simulink model "test_synchronous_machines_EMT_Phasor"  (R2025b)
settings: Solver=VariableStepAuto  StartTime=0.0  StopTime=20  RelTol=1e-3
undefined symbols (not defined in the file): Circuit, DiscIntNeverNeededParam, Open, Short
libraries: fl_lib x6, ee_lib_for_power_systems x6, ee_lib x6, nesl_utility x3
settings Model: Creator=gdudgeon  LastModifiedBy=gdudgeon
settings RTWCC: GPUComputeCapability=3.5

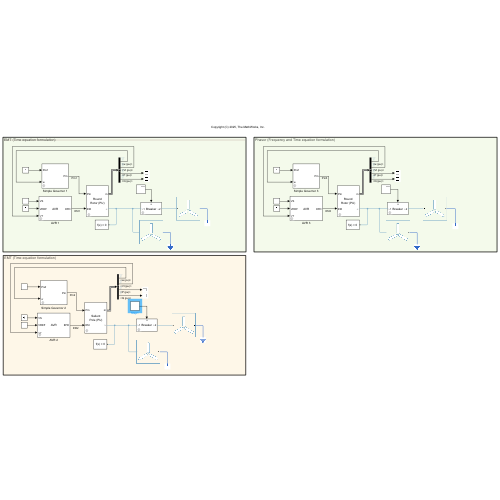
[thumbnail: Simulink's stored preview of the top-level diagram]
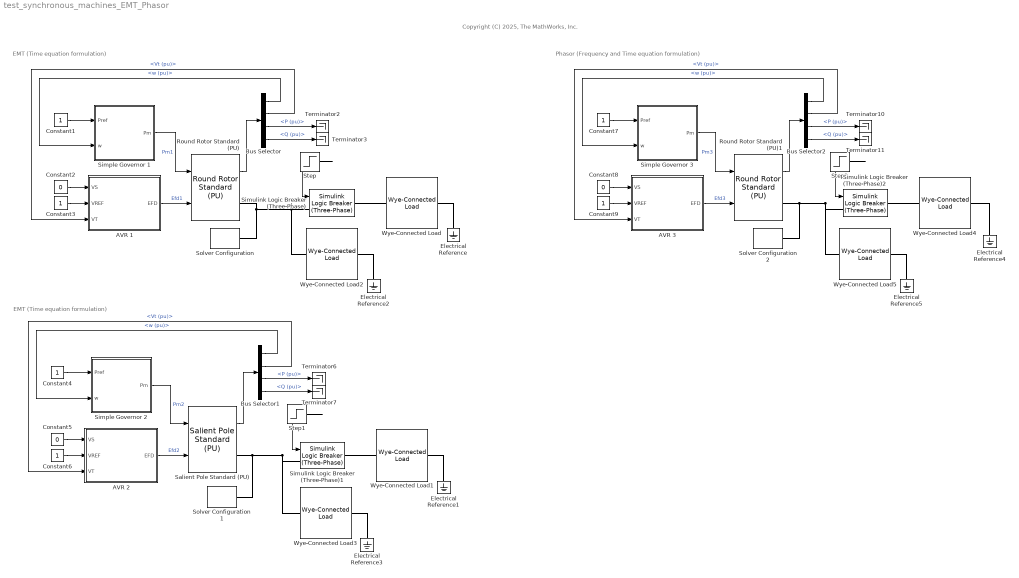
== system test_synchronous_machines_EMT_Phasor ==
  note: EMT (Time equation formulation)
  note: EMT (Time equation formulation)
  note: Phasor (Frequency and Time equation formulation)
  note: Copyright (C) 2025, The MathWorks, Inc.
  AVR 1 : Subsystem  mask{K=200, TE=0.05, EMIN=0, EMAX=4}
      mask Display: disp('AVR')
  AVR 2 : Subsystem  mask{K=200, TE=0.05, EMIN=0, EMAX=4}
      mask Display: disp('AVR')
  AVR 3 : Subsystem  mask{K=200, TE=0.05, EMIN=0, EMAX=4}
      mask Display: disp('AVR')
  Bus Selector : BusSelector  OutputSignals=w (pu),Vt (pu),P (pu),Q (pu)
  Bus Selector1 : BusSelector  OutputSignals=w (pu),Vt (pu),P (pu),Q (pu)
  Bus Selector2 : BusSelector  OutputSignals=w (pu),Vt (pu),P (pu),Q (pu)
  Constant{1,3..4,6..7,9} (6 alike) : Constant
  Constant2 : Constant  Value=0
  Constant5 : Constant  Value=0
  Constant8 : Constant  Value=0
  Electrical Reference{,1..5} (6 alike) : fl_lib/Electrical/Electrical Elements/Electrical Reference
  Round Rotor Standard (PU) : ee_lib_for_power_systems/Electromechanical Machines/Round Rotor Standard (PU)  Pnom=1e6  Vnom=20e3  Fnom=60  Xd=1.5  Xdp=0.4  Xdpp=0.25  Xq=1.4  Xqp=0.5  Xqpp=0.25  Xl=0.1  Ra=0.05  D_Q=[Short-Circuit Open-Circuit]  Tdp=1.2  Tdpp=0.05  Tdop=7  Tdopp=0.05  Tqp=1  Tqpp=0.05  Tqop=1  Tqopp=0.04  H=0.2  D=0  p=4
  Round Rotor Standard (PU)1 : ee_lib_for_power_systems/Electromechanical Machines/Round Rotor Standard (PU)  Pnom=1e6  Vnom=20e3  Fnom=60  Xd=1.5  Xdp=0.4  Xdpp=0.25  Xq=1.4  Xqp=0.5  Xqpp=0.25  Xl=0.1  Ra=0.05  D_Q=[Short-Circuit Open-Circuit]  Tdp=1.2  Tdpp=0.05  Tdop=7  Tdopp=0.05  Tqp=1  Tqpp=0.05  Tqop=1  Tqopp=0.04  H=0.2  D=0  p=4
  Salient Pole Standard (PU) : ee_lib_for_power_systems/Electromechanical Machines/Salient Pole Standard (PU)  Pnom=1e6  Vnom=20e3  Fnom=60  Xd=1.5  Xdp=0.4  Xdpp=0.25  Xq=1.4  Xqpp=0.25  Xl=0.1  Ra=0.05  D_Q=[Short-Circuit Open-Circuit]  Tdp=1.2  Tdpp=0.05  Tdop=7  Tdopp=0.05  Tqpp=0.05  Tqopp=0.04  H=0.2  D=0  p=4
  Simple Governor 1 : Subsystem  mask{R=0.05, T1=0.5, P_MAX=2, P_MIN=0}
  Simple Governor 2 : Subsystem  mask{R=0.05, T1=0.5, P_MAX=2, P_MIN=0}
  Simple Governor 3 : Subsystem  mask{R=0.05, T1=0.5, P_MAX=2, P_MIN=0}
  Simulink Logic Breaker (Three-Phase) : ee_lib_for_power_systems/Network Components/Simulink Logic Breaker (Three-Phase)  initB=1  Ron=1e-6  Goff=1e-6  Ts=5e-5
  Simulink Logic Breaker (Three-Phase)1 : ee_lib_for_power_systems/Network Components/Simulink Logic Breaker (Three-Phase)  initB=1  Ron=1e-6  Goff=1e-6  Ts=5e-5
  Simulink Logic Breaker (Three-Phase)2 : ee_lib_for_power_systems/Network Components/Simulink Logic Breaker (Three-Phase)  initB=1  Ron=1e-6  Goff=1e-6  Ts=5e-5
  "Solver Configuration " : nesl_utility/Solver Configuration  PhysicalDomain=network_engine_domain  SubClassName=solver  LeftPortType=input  RightPortType=generic  Tones=[]  Harmonics=[]  SimulateNoise=off  Profile=off  UseLocalSampling=off  EnableSwitchedLinearOptims=on  FrequencyDomain=off  UseCCode=off  RelTol=0.001  AbsTol=0.001  MinStep=1e-09  ToWorkspace=off  RevertToSquareIcSolve=off  NumHomotopyIterations=100  PhasorMode=off  PhasorModeNumHarmonics=1  ConsistencySolver=NEWTON_XTOL_AFTER_FTOL  IndexReductionMethod=None  DoDC=off  ResidualTolerance=1e-09  ConsistencyTolSource=GLOBAL  ConsistencyAbsTol=0.001  ConsistencyRelTol=0.001  ConsistencyTolFactor=0.001  UseLocalSolver=on  LocalSolverChoice=NE_PARTITIONING_ADVANCER  ResolveIndetEquations=off  FunctionEvalNumThread=1  LocalSolverSampleTime=50e-6  DoFixedCost=off  MaxNonlinIter=2  MaxModeIter=2  ComputeImpulses=off  ImpulseIterations=2  LinearAlgebra=Sparse  LinearAlgebraNumThread=0  EquationFormulation=NE_TIME_EF  DelaysMemoryBudget=1024  AutomaticFiltering=off  FilteringTimeConstant=0.001  PartitionStorageMethod=AS_NEEDED  PartitionMemoryBudget=1024  PartitionMethod=ROBUST  MultibodyUseLocalSolver=off  MultibodyLocalSolverChoice=ODE1  MultibodyLocalSolverSampleTime=0.001
  Solver Configuration 1 : nesl_utility/Solver Configuration  PhysicalDomain=network_engine_domain  SubClassName=solver  LeftPortType=input  RightPortType=generic  Tones=[]  Harmonics=[]  SimulateNoise=off  Profile=off  UseLocalSampling=off  EnableSwitchedLinearOptims=on  FrequencyDomain=off  UseCCode=off  RelTol=0.001  AbsTol=0.001  MinStep=1e-09  ToWorkspace=off  RevertToSquareIcSolve=off  NumHomotopyIterations=100  PhasorMode=off  PhasorModeNumHarmonics=1  ConsistencySolver=NEWTON_XTOL_AFTER_FTOL  IndexReductionMethod=None  DoDC=off  ResidualTolerance=1e-09  ConsistencyTolSource=GLOBAL  ConsistencyAbsTol=0.001  ConsistencyRelTol=0.001  ConsistencyTolFactor=0.001  UseLocalSolver=on  LocalSolverChoice=NE_PARTITIONING_ADVANCER  ResolveIndetEquations=off  FunctionEvalNumThread=1  LocalSolverSampleTime=50e-6  DoFixedCost=off  MaxNonlinIter=2  MaxModeIter=2  ComputeImpulses=off  ImpulseIterations=2  LinearAlgebra=Sparse  LinearAlgebraNumThread=0  EquationFormulation=NE_TIME_EF  DelaysMemoryBudget=1024  AutomaticFiltering=off  FilteringTimeConstant=0.001  PartitionStorageMethod=AS_NEEDED  PartitionMemoryBudget=1024  PartitionMethod=ROBUST  MultibodyUseLocalSolver=off  MultibodyLocalSolverChoice=ODE1  MultibodyLocalSolverSampleTime=0.001
  Solver Configuration 2 : nesl_utility/Solver Configuration  PhysicalDomain=network_engine_domain  SubClassName=solver  LeftPortType=input  RightPortType=generic  Tones=[]  Harmonics=[]  SimulateNoise=off  Profile=off  UseLocalSampling=off  EnableSwitchedLinearOptims=on  FrequencyDomain=off  UseCCode=off  RelTol=0.001  AbsTol=0.001  MinStep=1e-09  ToWorkspace=off  RevertToSquareIcSolve=off  NumHomotopyIterations=100  PhasorMode=off  PhasorModeNumHarmonics=1  ConsistencySolver=NEWTON_XTOL_AFTER_FTOL  IndexReductionMethod=None  DoDC=off  ResidualTolerance=1e-09  ConsistencyTolSource=GLOBAL  ConsistencyAbsTol=0.001  ConsistencyRelTol=0.001  ConsistencyTolFactor=0.001  UseLocalSolver=on  LocalSolverChoice=NE_BACKWARD_EULER_ADVANCER  ResolveIndetEquations=off  FunctionEvalNumThread=1  LocalSolverSampleTime=1/120  DoFixedCost=on  MaxNonlinIter=2  MaxModeIter=2  ComputeImpulses=off  ImpulseIterations=2  LinearAlgebra=auto  LinearAlgebraNumThread=0  EquationFormulation=NE_FREQUENCY_TIME_EF  DelaysMemoryBudget=1024  AutomaticFiltering=off  FilteringTimeConstant=0.001  PartitionStorageMethod=AS_NEEDED  PartitionMemoryBudget=1024  PartitionMethod=ROBUST  MultibodyUseLocalSolver=off  MultibodyLocalSolverChoice=ODE1  MultibodyLocalSolverSampleTime=0.001
  Step : Step  Time=10  SampleTime=5e-5
  Step1 : Step  Time=10  SampleTime=5e-5
  Step2 : Step  Time=10  SampleTime=5e-5
  Terminator{2..3,6..7,10..11} (6 alike) : Terminator
  Wye-Connected Load{,1..5} (6 alike) : ee_lib/Passive/RLC Assemblies/Wye-Connected Load  port_option=ee.enum.threePhasePort.composite  parameterization=ee.enum.rlc.parameterization.ratedpower  component_structure=ee.enum.rlc.structure.R  component_structure_PQ=ee.enum.rlc.structure.R  R=1 Ohm  L=1e-3 H  C=1e-6 F  VRated=20e3 V  FRated=60 Hz  P=5e5 W  Qpos=3e5 A*V  Qneg=-1e2 A*V  R_parasitic=0 Ohm  G_parasitic=0 1/Ohm  R_parasitic_PQ=0 Ohm  G_parasitic_PQ=0 1/Ohm  Vmag0=24e3 V  Vang0=0 deg  Freq0=60 Hz  IL_specify=off  IL_priority=High  IL=[0, 0, 0] A  IL_nominal_specify=off  IL_nominal_value=1  IL_nominal_unit=A  VC_specify=off  VC_priority=High  VC=[0, 0, 0] V  VC_nominal_specify=off  VC_nominal_value=1  VC_nominal_unit=V
  wires:
  Round Rotor Standard (PU)/1 -> Bus Selector/1
  AVR 1/1(EFD) -> Round Rotor Standard (PU)/2  "Efd1"
  Simple Governor 1/1(Pm) -> Round Rotor Standard (PU)/1  "Pm1"
  Step/1 -> Simulink Logic Breaker (Three-Phase)/1
  Bus Selector/1 -> Simple Governor 1/2(w)  "<w (pu)>"
  Constant1/1 -> Simple Governor 1/1(Pref)
  Bus Selector/2 -> AVR 1/3(VT)  "<Vt (pu)>"
  Constant3/1 -> AVR 1/2(VREF)
  Constant2/1 -> AVR 1/1(VS)
  Bus Selector/3 -> Terminator2/1  "<P (pu)>"
  Bus Selector/4 -> Terminator3/1  "<Q (pu)>"
  Bus Selector1/4 -> Terminator7/1  "<Q (pu)>"
  Bus Selector1/3 -> Terminator6/1  "<P (pu)>"
  Constant5/1 -> AVR 2/1(VS)
  Constant6/1 -> AVR 2/2(VREF)
  Bus Selector1/2 -> AVR 2/3(VT)  "<Vt (pu)>"
  Constant4/1 -> Simple Governor 2/1(Pref)
  Bus Selector1/1 -> Simple Governor 2/2(w)  "<w (pu)>"
  Step1/1 -> Simulink Logic Breaker (Three-Phase)1/1
  Simple Governor 2/1(Pm) -> Salient Pole Standard (PU)/1  "Pm2"
  AVR 2/1(EFD) -> Salient Pole Standard (PU)/2  "Efd2"
  Salient Pole Standard (PU)/1 -> Bus Selector1/1
  Bus Selector2/4 -> Terminator11/1  "<Q (pu)>"
  Bus Selector2/3 -> Terminator10/1  "<P (pu)>"
  Constant8/1 -> AVR 3/1(VS)
  Constant9/1 -> AVR 3/2(VREF)
  Bus Selector2/2 -> AVR 3/3(VT)  "<Vt (pu)>"
  Constant7/1 -> Simple Governor 3/1(Pref)
  Bus Selector2/1 -> Simple Governor 3/2(w)  "<w (pu)>"
  Simple Governor 3/1(Pm) -> Round Rotor Standard (PU)1/1  "Pm3"
  AVR 3/1(EFD) -> Round Rotor Standard (PU)1/2  "Efd3"
  Round Rotor Standard (PU)1/1 -> Bus Selector2/1
  Step2/1 -> Simulink Logic Breaker (Three-Phase)2/1
  connections:
  Simulink Logic Breaker (Three-Phase)/LConn1 -- Round Rotor Standard (PU)/RConn1 -- "Solver Configuration "/RConn1 -- Wye-Connected Load2/LConn1
  Electrical Reference/LConn1 -- Wye-Connected Load/RConn1
  Simulink Logic Breaker (Three-Phase)/RConn1 -- Wye-Connected Load/LConn1
  Simulink Logic Breaker (Three-Phase)1/RConn1 -- Wye-Connected Load1/LConn1
  Electrical Reference1/LConn1 -- Wye-Connected Load1/RConn1
  Solver Configuration 1/RConn1 -- Simulink Logic Breaker (Three-Phase)1/LConn1 -- Wye-Connected Load3/LConn1 -- Salient Pole Standard (PU)/RConn1
  Electrical Reference2/LConn1 -- Wye-Connected Load2/RConn1
  Electrical Reference3/LConn1 -- Wye-Connected Load3/RConn1
  Electrical Reference5/LConn1 -- Wye-Connected Load5/RConn1
  Electrical Reference4/LConn1 -- Wye-Connected Load4/RConn1
  Simulink Logic Breaker (Three-Phase)2/RConn1 -- Wye-Connected Load4/LConn1
  Round Rotor Standard (PU)1/RConn1 -- Solver Configuration 2/RConn1 -- Simulink Logic Breaker (Three-Phase)2/LConn1 -- Wye-Connected Load5/LConn1

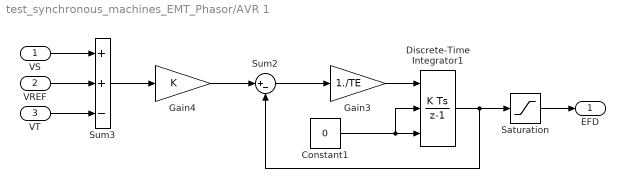
== system test_synchronous_machines_EMT_Phasor/AVR 1 ==
  VS : Inport
  VREF : Inport  Port=2
  VT : Inport  Port=3
  Constant1 : Constant  Value=0  SampleTime=-1
  Discrete-Time Integrator1 : DiscreteIntegrator  ExternalReset=rising  InitialConditionSource=external  SampleTime=-1  UpperSaturationLimit=EMAX  LowerSaturationLimit=EMIN  ICPrevOutput=DiscIntNeverNeededParam  ICPrevScaledInput=DiscIntNeverNeededParam
  Gain3 : Gain  Gain=1./TE
  Gain4 : Gain  Gain=K
  Saturation : Saturate  UpperLimit=EMAX  LowerLimit=EMIN
  Sum2 : Sum  Inputs=|+-
  Sum3 : Sum  Inputs=++-
  EFD : Outport
  wires:
  Sum3/1 -> Gain4/1
  Discrete-Time Integrator1/1 -> Saturation/1, Sum2/2
  Constant1/1 -> Discrete-Time Integrator1/2, Discrete-Time Integrator1/3
  Gain3/1 -> Discrete-Time Integrator1/1
  Sum2/1 -> Gain3/1
  Gain4/1 -> Sum2/1
  VT/1 -> Sum3/3
  VREF/1 -> Sum3/2
  VS/1 -> Sum3/1
  Saturation/1 -> EFD/1

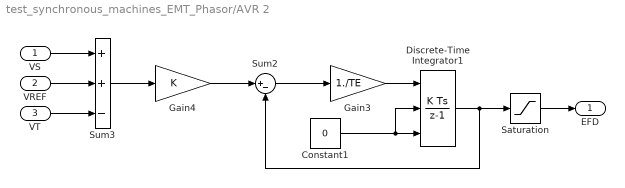
== system test_synchronous_machines_EMT_Phasor/AVR 2 ==
  VS : Inport
  VREF : Inport  Port=2
  VT : Inport  Port=3
  Constant1 : Constant  Value=0  SampleTime=-1
  Discrete-Time Integrator1 : DiscreteIntegrator  ExternalReset=rising  InitialConditionSource=external  SampleTime=-1  UpperSaturationLimit=EMAX  LowerSaturationLimit=EMIN  ICPrevOutput=DiscIntNeverNeededParam  ICPrevScaledInput=DiscIntNeverNeededParam
  Gain3 : Gain  Gain=1./TE
  Gain4 : Gain  Gain=K
  Saturation : Saturate  UpperLimit=EMAX  LowerLimit=EMIN
  Sum2 : Sum  Inputs=|+-
  Sum3 : Sum  Inputs=++-
  EFD : Outport
  wires:
  Saturation/1 -> EFD/1
  VS/1 -> Sum3/1
  VREF/1 -> Sum3/2
  VT/1 -> Sum3/3
  Gain4/1 -> Sum2/1
  Sum2/1 -> Gain3/1
  Gain3/1 -> Discrete-Time Integrator1/1
  Constant1/1 -> Discrete-Time Integrator1/3, Discrete-Time Integrator1/2
  Discrete-Time Integrator1/1 -> Sum2/2, Saturation/1
  Sum3/1 -> Gain4/1

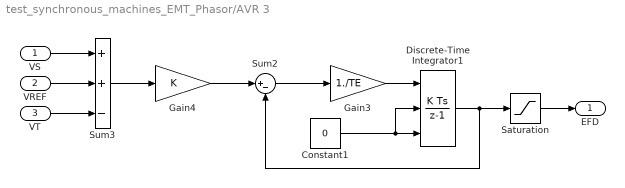
== system test_synchronous_machines_EMT_Phasor/AVR 3 ==
  VS : Inport
  VREF : Inport  Port=2
  VT : Inport  Port=3
  Constant1 : Constant  Value=0  SampleTime=-1
  Discrete-Time Integrator1 : DiscreteIntegrator  ExternalReset=rising  InitialConditionSource=external  SampleTime=-1  UpperSaturationLimit=EMAX  LowerSaturationLimit=EMIN  ICPrevOutput=DiscIntNeverNeededParam  ICPrevScaledInput=DiscIntNeverNeededParam
  Gain3 : Gain  Gain=1./TE
  Gain4 : Gain  Gain=K
  Saturation : Saturate  UpperLimit=EMAX  LowerLimit=EMIN
  Sum2 : Sum  Inputs=|+-
  Sum3 : Sum  Inputs=++-
  EFD : Outport
  wires:
  Sum3/1 -> Gain4/1
  Discrete-Time Integrator1/1 -> Saturation/1, Sum2/2
  Constant1/1 -> Discrete-Time Integrator1/2, Discrete-Time Integrator1/3
  Gain3/1 -> Discrete-Time Integrator1/1
  Sum2/1 -> Gain3/1
  Gain4/1 -> Sum2/1
  VT/1 -> Sum3/3
  VREF/1 -> Sum3/2
  VS/1 -> Sum3/1
  Saturation/1 -> EFD/1

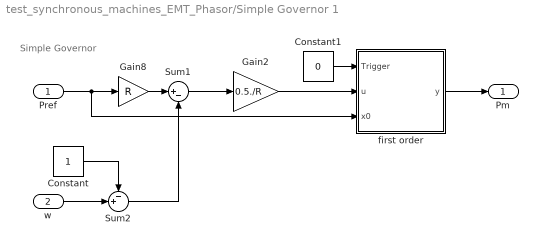
== system test_synchronous_machines_EMT_Phasor/Simple Governor 1 ==
  note: Simple Governor
  Pref : Inport
  w : Inport  Port=2
  Constant : Constant  SampleTime=-1
  Constant1 : Constant  Value=0  SampleTime=-1
  Gain2 : Gain  Gain=0.5./R
  Gain8 : Gain  Gain=R
  Sum1 : Sum  Inputs=|+-
  Sum2 : Sum  Inputs=-+|
  first order : Subsystem
      mask Display: fprintf('1\n------------\n1 + T1s');
  Pm : Outport
  wires:
  Sum1/1 -> Gain2/1
  Pref/1 -> first order/3(x0), Gain8/1
  Constant/1 -> Sum2/1
  Sum2/1 -> Sum1/2
  Gain8/1 -> Sum1/1
  Gain2/1 -> first order/2(u)
  w/1 -> Sum2/2
  first order/1(y) -> Pm/1
  Constant1/1 -> first order/1(Trigger)

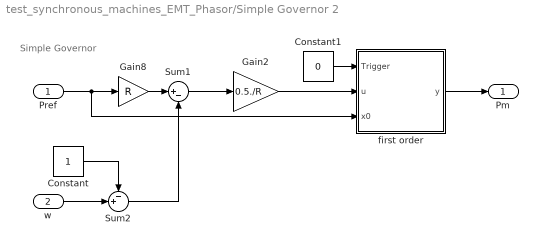
== system test_synchronous_machines_EMT_Phasor/Simple Governor 2 ==
  note: Simple Governor
  Pref : Inport
  w : Inport  Port=2
  Constant : Constant  SampleTime=-1
  Constant1 : Constant  Value=0  SampleTime=-1
  Gain2 : Gain  Gain=0.5./R
  Gain8 : Gain  Gain=R
  Sum1 : Sum  Inputs=|+-
  Sum2 : Sum  Inputs=-+|
  first order : Subsystem
      mask Display: fprintf('1\n------------\n1 + T1s');
  Pm : Outport
  wires:
  Constant1/1 -> first order/1(Trigger)
  first order/1(y) -> Pm/1
  w/1 -> Sum2/2
  Gain2/1 -> first order/2(u)
  Gain8/1 -> Sum1/1
  Sum2/1 -> Sum1/2
  Constant/1 -> Sum2/1
  Pref/1 -> Gain8/1, first order/3(x0)
  Sum1/1 -> Gain2/1

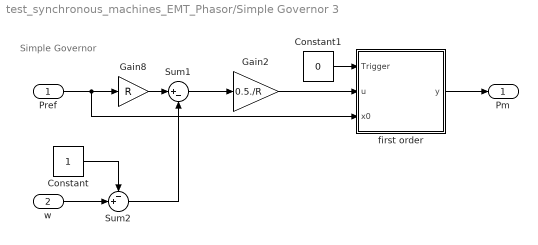
== system test_synchronous_machines_EMT_Phasor/Simple Governor 3 ==
  note: Simple Governor
  Pref : Inport
  w : Inport  Port=2
  Constant : Constant  SampleTime=-1
  Constant1 : Constant  Value=0  SampleTime=-1
  Gain2 : Gain  Gain=0.5./R
  Gain8 : Gain  Gain=R
  Sum1 : Sum  Inputs=|+-
  Sum2 : Sum  Inputs=-+|
  first order : Subsystem
      mask Display: fprintf('1\n------------\n1 + T1s');
  Pm : Outport
  wires:
  Sum1/1 -> Gain2/1
  Pref/1 -> first order/3(x0), Gain8/1
  Constant/1 -> Sum2/1
  Sum2/1 -> Sum1/2
  Gain8/1 -> Sum1/1
  Gain2/1 -> first order/2(u)
  w/1 -> Sum2/2
  first order/1(y) -> Pm/1
  Constant1/1 -> first order/1(Trigger)

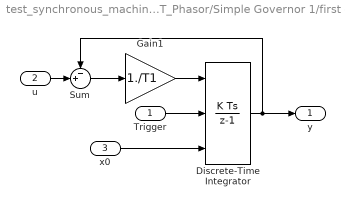
== system test_synchronous_machines_EMT_Phasor/Simple Governor 1/first order ==
  Trigger : Inport
  u : Inport  Port=2
  x0 : Inport  Port=3
  Discrete-Time Integrator : DiscreteIntegrator  ExternalReset=rising  InitialConditionSource=external  SampleTime=-1  LimitOutput=on  UpperSaturationLimit=P_MAX  LowerSaturationLimit=P_MIN  ICPrevOutput=DiscIntNeverNeededParam  ICPrevScaledInput=DiscIntNeverNeededParam
  Gain1 : Gain  Gain=1./T1
  Sum : Sum  Inputs=-+|
  y : Outport
  wires:
  Trigger/1 -> Discrete-Time Integrator/2
  u/1 -> Sum/2
  Sum/1 -> Gain1/1
  x0/1 -> Discrete-Time Integrator/3
  Discrete-Time Integrator/1 -> y/1, Sum/1
  Gain1/1 -> Discrete-Time Integrator/1

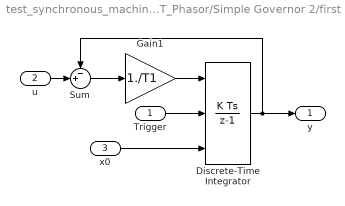
== system test_synchronous_machines_EMT_Phasor/Simple Governor 2/first order ==
  Trigger : Inport
  u : Inport  Port=2
  x0 : Inport  Port=3
  Discrete-Time Integrator : DiscreteIntegrator  ExternalReset=rising  InitialConditionSource=external  SampleTime=-1  LimitOutput=on  UpperSaturationLimit=P_MAX  LowerSaturationLimit=P_MIN  ICPrevOutput=DiscIntNeverNeededParam  ICPrevScaledInput=DiscIntNeverNeededParam
  Gain1 : Gain  Gain=1./T1
  Sum : Sum  Inputs=-+|
  y : Outport
  wires:
  Gain1/1 -> Discrete-Time Integrator/1
  Discrete-Time Integrator/1 -> Sum/1, y/1
  x0/1 -> Discrete-Time Integrator/3
  Sum/1 -> Gain1/1
  u/1 -> Sum/2
  Trigger/1 -> Discrete-Time Integrator/2

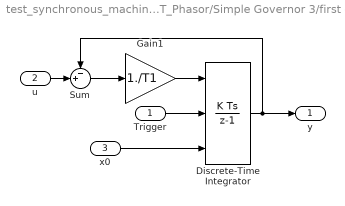
== system test_synchronous_machines_EMT_Phasor/Simple Governor 3/first order ==
  Trigger : Inport
  u : Inport  Port=2
  x0 : Inport  Port=3
  Discrete-Time Integrator : DiscreteIntegrator  ExternalReset=rising  InitialConditionSource=external  SampleTime=-1  LimitOutput=on  UpperSaturationLimit=P_MAX  LowerSaturationLimit=P_MIN  ICPrevOutput=DiscIntNeverNeededParam  ICPrevScaledInput=DiscIntNeverNeededParam
  Gain1 : Gain  Gain=1./T1
  Sum : Sum  Inputs=-+|
  y : Outport
  wires:
  Trigger/1 -> Discrete-Time Integrator/2
  u/1 -> Sum/2
  Sum/1 -> Gain1/1
  x0/1 -> Discrete-Time Integrator/3
  Discrete-Time Integrator/1 -> y/1, Sum/1
  Gain1/1 -> Discrete-Time Integrator/1
